simulink model "bouncing_ball_continuous"  (R2022b)
settings: Solver=VariableStepAuto  StartTime=0.0  StopTime=10.0  RelTol=1e-3
settings Model: Creator=user  LastModifiedBy=user

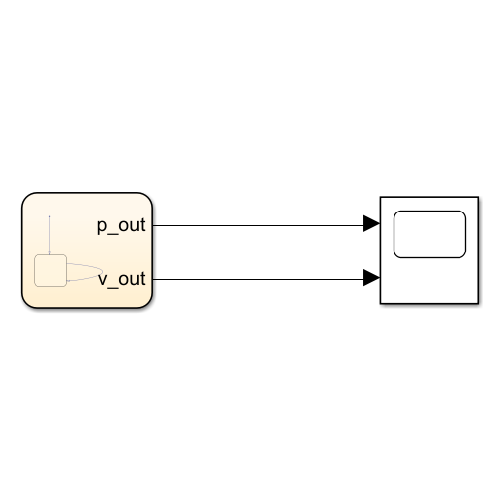
[thumbnail: Simulink's stored preview of the top-level diagram]
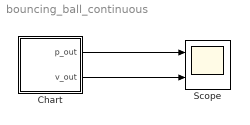
== system bouncing_ball_continuous ==
  Chart : Stateflow chart  TreatAsAtomicUnit=on
  Scope : Scope  NumInputPorts=2
  wires:
  Chart/2(v_out) -> Scope/2
  Chart/1(p_out) -> Scope/1

== stateflow chart bouncing_ball_continuous/Chart ==
  settings: updateMethod=CONTINUOUS
  state Falling
    du:
    p_dot = v;
    v_dot = -9.81;
    p_out = p;
    v_out = v;
  (default) -> Falling : {
      | p = 10;
      | v = 15;
      | }
  Falling -> Falling : [p <= 0 && v < 0]
      | {
      | p = 0;
      | v = -0.8*v;
      | }
  data: p local; v local; p_out output; v_out output
  data p settings: updateMethod=SF_CONTINUOUS_TIME_DATA
  data v settings: updateMethod=SF_CONTINUOUS_TIME_DATA
